simulink model "closeloopPendulum"  (R2021b)
settings: Solver=VariableStepAuto  StartTime=0.0  StopTime=40  RelTol=1e-3
values from neighbouring files (symbols this model uses):
  b = 0.1    [VariablesDelSistema.m]
  denC = cell2mat(den)    [VariablesDelSistema.m]
  denCcarrito = cell2mat(dencarrito)    [VariablesDelSistema.m]
  g = -9.81    [VariablesDelSistema.m]
  I = 0.006    [VariablesDelSistema.m]
  L = 0.5 + 0.1*8    (= 1.3)    [VariablesDelSistema.m]
  m = 0.2    [VariablesDelSistema.m]
  M = 0.5 + 0.1*7    (= 1.2)    [VariablesDelSistema.m]
  numC = cell2mat(num)    [VariablesDelSistema.m]
  numCcarrito = cell2mat(numcarrito)    [VariablesDelSistema.m]
  T = 1 / Fmuestreo    [VariablesDelSistema.m]
settings Model: Creator=jualc  LastModifiedBy=e.delpico.2020

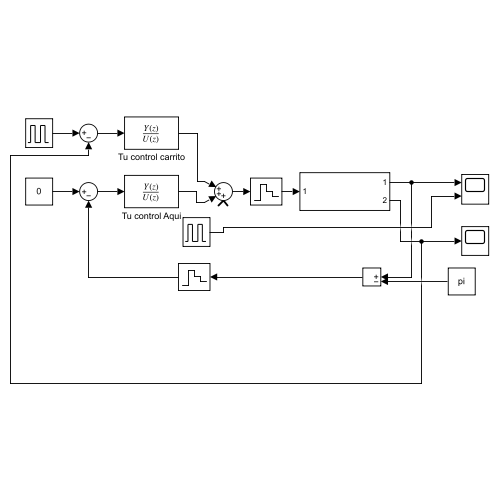
[thumbnail: Simulink's stored preview of the top-level diagram]
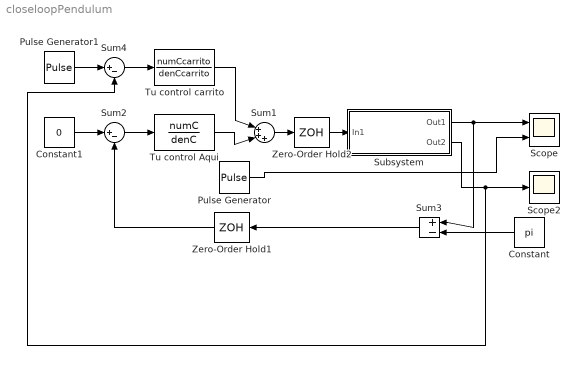
== system closeloopPendulum ==
  Constant : Constant  Value=pi
  Constant1 : Constant  Value=0
  Pulse Generator : DiscretePulseGenerator  PulseType=Time based  Amplitude=100  PulseWidth=0.1
  Pulse Generator1 : DiscretePulseGenerator  PulseType=Time based  Period=20  PulseWidth=50
  Scope : Scope  NumInputPorts=2
  Scope2 : Scope
  Subsystem : Subsystem
  Sum1 : Sum  Inputs=|+++
  Sum2 : Sum  Inputs=|+-
  Sum3 : Sum  Inputs=|+-
  Sum4 : Sum  Inputs=|+-
  Tu control Aqui : DiscreteTransferFcn  Numerator=numC  Denominator=denC  SampleTime=T
  Tu control carrito : DiscreteTransferFcn  Numerator=numCcarrito  Denominator=denCcarrito  SampleTime=T
  Zero-Order Hold1 : ZeroOrderHold  SampleTime=T
  Zero-Order Hold2 : ZeroOrderHold  SampleTime=T
  wires:
  Subsystem/1(Out1) -> Sum3/1, Scope/1
  Subsystem/2(Out2) -> Scope2/1, Sum4/2
  Constant/1 -> Sum3/2
  Sum3/1 -> Zero-Order Hold1/1
  Sum2/1 -> Tu control Aqui/1
  Zero-Order Hold1/1 -> Sum2/2
  Constant1/1 -> Sum2/1
  Pulse Generator/1 -> Scope/2
  Sum1/1 -> Zero-Order Hold2/1
  Zero-Order Hold2/1 -> Subsystem/1(In1)
  Sum4/1 -> Tu control carrito/1
  Pulse Generator1/1 -> Sum4/1
  Tu control Aqui/1 -> Sum1/2
  Tu control carrito/1 -> Sum1/1

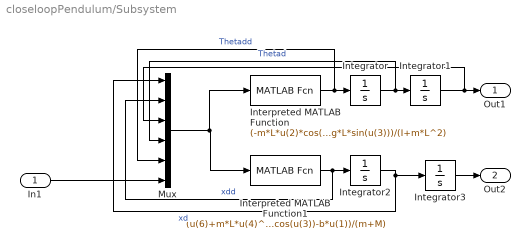
== system closeloopPendulum/Subsystem ==
  In1 : Inport
  Integrator : Integrator
  Integrator1 : Integrator  InitialCondition=pi
  Integrator2 : Integrator
  Integrator3 : Integrator
  Interpreted MATLAB Function : MATLABFcn  MATLABFcn=(-m*L*u(2)*cos(u(3))-m*g*L*sin(u(3)))/(I+m*L^2)
  Interpreted MATLAB Function1 : MATLABFcn  MATLABFcn=(u(6)+m*L*u(4)^2*sin(u(3))-m*L*u(5)*cos(u(3))-b*u(1))/(m+M)
  Mux : Mux  Inputs=6
  Out1 : Outport
  Out2 : Outport  Port=2
  wires:
  Integrator/1 -> Mux/4, Integrator1/1  "Thetad"
  Interpreted MATLAB Function1/1 -> Mux/2, Integrator2/1  "xdd"
  Integrator2/1 -> Integrator3/1, Mux/1  "xd"
  Mux/1 -> Interpreted MATLAB Function/1, Interpreted MATLAB Function1/1
  Integrator1/1 -> Out1/1, Mux/3
  In1/1 -> Mux/6
  Interpreted MATLAB Function/1 -> Mux/5, Integrator/1  "Thetadd"
  Integrator3/1 -> Out2/1
